simulink model "Simulacion_lineal_punto_d"  (R2021a)
settings: Solver=VariableStepAuto  StartTime=0.0  StopTime=10.0  RelTol=1e-3
settings Model: Creator=mateo  LastModifiedBy=mateo

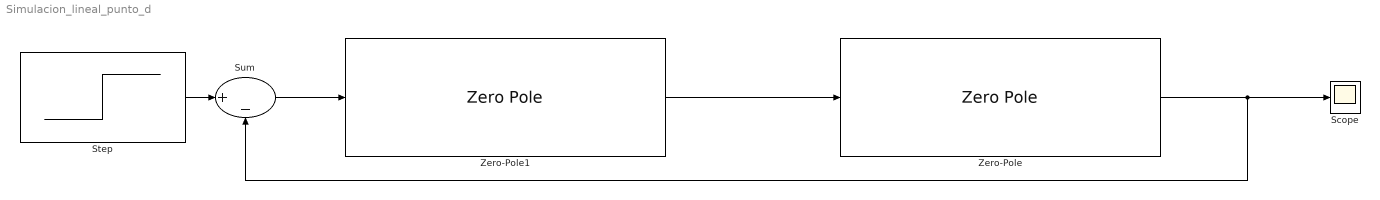
== system Simulacion_lineal_punto_d ==
  Scope : Scope
  Step : Step  SampleTime=0
  Sum : Sum  Inputs=|+-
  Zero-Pole : ZeroPole  Zeros=[2.2904e+03]  Poles=[3.04 -3.29 -2.2904e+03]  Gain=[2.5]
  Zero-Pole1 : ZeroPole  Zeros=[-3.04 -3.29]  Poles=[0 -100000]  Gain=[-3.9811e+06]
  wires:
  Zero-Pole1/1 -> Zero-Pole/1
  Zero-Pole/1 -> Sum/2, Scope/1
  Sum/1 -> Zero-Pole1/1
  Step/1 -> Sum/1
